simulink model "MotionLab_DigitalTwin"  (R2024b)
settings: Solver=ode3  StartTime=0.0  StopTime=inf  FixedStep=Ts  RelTol=1e-3  AbsTol=1e-3
model workspace: external: MATLAB File .\Parameters.m (data not in the file)
values from neighbouring files (symbols this model uses):
  L2 = 830e-3    (= 0.83)    [Robot_parameters.m]
  L3 = 1160e-3    (= 1.16)    [Robot_parameters.m]
  L4 = 250e-3    (= 0.25)    [Robot_parameters.m]
undefined symbols (not defined in the file or in its folder): smiData, smiDataBig, smiDataBigTop, smiDataRobot, Var, X, Y, Z
libraries: sm_lib x490, nesl_utility x87, slrealtimeutilitieslib x1, slrealtimeiplib x1, aerolibanimutils x1
(part 1 of 15)
settings Model: SimulationMode=accelerator  Creator=thoma  LastModifiedBy=jojoa
settings SolverCC: AutoScaleAbsTol=off  AlgebraicLoopSolver=TrustRegion  MaxZcPerStep=1
settings DebuggingCC: UnconnectedInputMsg=warning  UnconnectedOutputMsg=warning  UnconnectedLineMsg=warning  SymbolicDimsDataTypeCodeGenerationDiagnostic=none
settings ModelReferenceCC: EnableRefExpFcnMdlSchedulingChecks=on
settings SFSimCC: CustomCodeUndefinedFunction=UseInterfaceOnly
settings RTWCC: GPUComputeCapability=3.5  DLArmComputeVersion=19.05
settings SimscapeCC: SimscapeLogType=all  SimscapeLogSimulationStatistics=on  SimscapeLogDataHistory=10000
settings ExplorerConfigSet: InternalSimMechanicsExplorerSettings="<ExplorerConfiguration><canonicalview>default</canonicalview><AnimationSetting><BasePlaybackSpeed>1.0</BasePlaybackSpeed><PlaybackSpeedFactor>1.0</PlaybackSpeedFactor></AnimationSetting><TilePanel><TileInfo><Tiles Columns=\"1\" Count=\"1\" Rows=\"1\"><Column Weight=\"1\"/><Row Weight=\"1\"/><Tile Height=\"1\" Width=\"1\" X=\"0\" Y=\"0\"/></Tiles></TileInfo><SceneInfo><SceneViewer><BGColor><R>1</R><G>1</G><B>1</B></BGColor><Camera><DoPerspective>off</DoPerspective><Position><X>-13.1233061332893666</X><Y>-1.45430535142352291</Y><Z>4.06844865702874081</Z></Position><Center><X>-0.172917730343304044</X><Y>1.29106577544240819</Y><Z>3.17239564313608469</Z></Center><Up><X>0.0683722661013297928</X><Y>0.00309773406366908866</Y><Z>0.997655069285893203</Z></Up><ViewLimDist>1</ViewLimDist><YLim>5.21326136870264634</YLim><XLim>6.07904176706880239</XLim></Camera></SceneViewer></SceneInfo></TilePanel><MechEditorPanel><Cameras/><GfxPanelCameraMap/><VideoCreator><PlaybackSpeedRatio>1.0</PlaybackSpeedRatio><FrameRate>30</FrameRate><VideoFormat>Motion JPEG AVI</VideoFormat><FrameSize>auto</FrameSize></VideoCreator></MechEditorPanel></ExplorerConfiguration>"

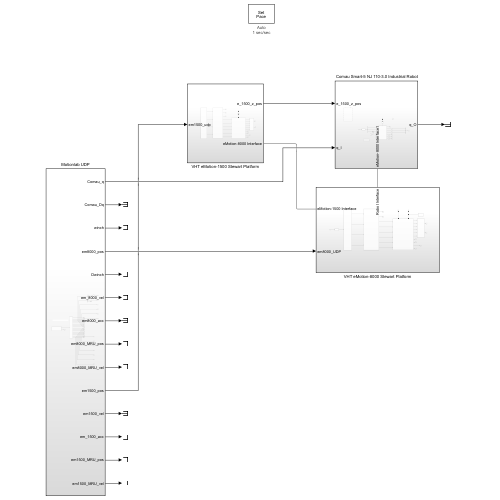
[thumbnail: Simulink's stored preview of the top-level diagram]
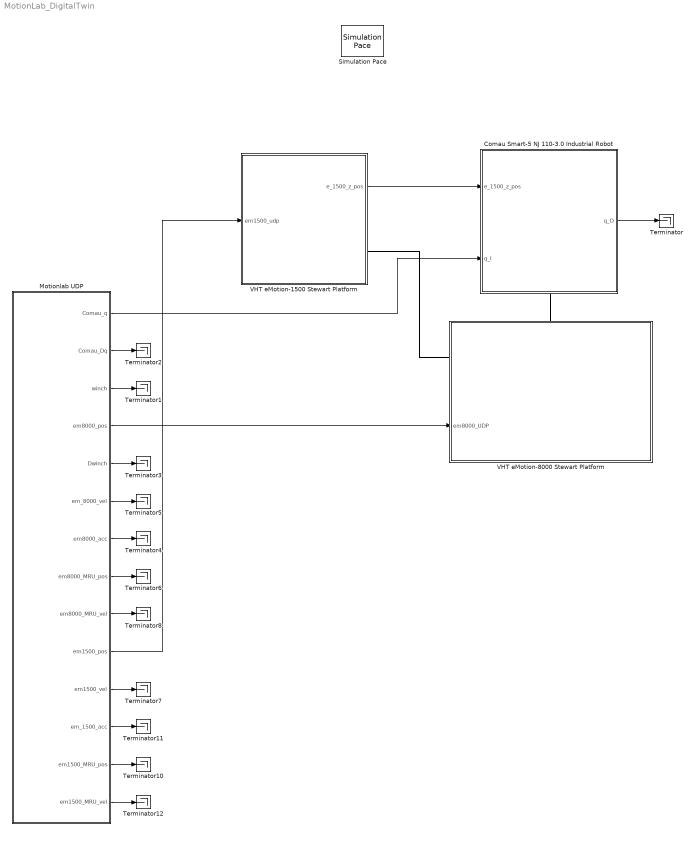
== system MotionLab_DigitalTwin ==
  " Comau Smart-5 NJ 110-3.0 Industrial Robot" : Subsystem
      settings: PortSchema="{\"entries\":[{\"content\":{\"sides\":[{\"content\":{\"connectorIds\":[\"In1\",\"In2\"]},\"type\":\"ConnectorPlacement.EquallySpacedRectSide\",\"uuid\":\"640b4a80-a183-4fda-808f-40bbc59803ff\"},{\"content\":{\"connectorIds\":[\"Out1\"],\"side\":\"RIGHT\"},\"type\":\"ConnectorPlacement.EquallySpacedRectSide\",\"uuid\":\"26bc9ede-0f7e-4968-8fcb-4700031f2d04\"},{\"content\":{\"side\":\"TOP\"},\"type\":\"ConnectorPlacement.EquallySpacedRectSide\",\"uuid\":\"f8c1678d-f904-4b2c-ba65-fdabdde128e7\"},{\"content\":{\"connectorIds\":[\"RConn1\"],\"side\":\"BOTTOM\"},\"type\":\"ConnectorPlacement.EquallySpacedRectSide\",\"uuid\":\"31ccf5cf-cde0-4868-907a-e8310ac905dd\"}]},\"type\":\"ConnectorPlacement.EquallySpacedConnector\",\"uuid\":\"53f72707-ebf3-419b-a015-bfc27a2c6f75\"}],\"packageUris\":[\"http://schema.mathworks.com/mf0/Connector/R2020b\"],\"version\":\"1.0\"}"
  Motionlab UDP : Subsystem
  Simulation Pace : aerolibanimutils/Simulation Pace  SimulationPace=1  SleepMode=Auto  OutputPaceError=off  SampleTime=0.1
  Terminator{,1..8,10..12} (12 alike) : Terminator
  VHT eMotion-1500 Stewart Platform : Subsystem
  VHT eMotion-8000 Stewart Platform : Subsystem
      settings: PortSchema="{\"entries\":[{\"content\":{\"sides\":[{\"content\":{\"connectorIds\":[\"LConn1\",\"In1\"]},\"type\":\"ConnectorPlacement.EquallySpacedRectSide\",\"uuid\":\"db0806e8-caa2-421d-936b-a6f75aa8bfb7\"},{\"content\":{\"side\":\"RIGHT\"},\"type\":\"ConnectorPlacement.EquallySpacedRectSide\",\"uuid\":\"91c2d1eb-1633-461d-b983-e6d74b9ad515\"},{\"content\":{\"connectorIds\":[\"LConn2\"],\"side\":\"TOP\"},\"type\":\"ConnectorPlacement.EquallySpacedRectSide\",\"uuid\":\"8a695272-575a-45c8-aed2-3cc82643c7b5\"}]},\"type\":\"ConnectorPlacement.EquallySpacedConnector\",\"uuid\":\"60269924-cfd7-445e-9c1f-e8fc9453bc0f\"}],\"packageUris\":[\"http://schema.mathworks.com/mf0/Connector/R2020b\"],\"version\":\"1.0\"}"
  wires:
  Motionlab UDP/2(Comau_Dq) -> Terminator2/1
  Motionlab UDP/3(winch) -> Terminator1/1
  VHT eMotion-1500 Stewart Platform/1(e_1500_z_pos) -> " Comau Smart-5 NJ 110-3.0 Industrial Robot"/1(e_1500_z_pos)
  Motionlab UDP/4(em8000_pos) -> VHT eMotion-8000 Stewart Platform/1(em8000_UDP)
  Motionlab UDP/1(Comau_q) -> " Comau Smart-5 NJ 110-3.0 Industrial Robot"/2(q_I)
  Motionlab UDP/14(em1500_MRU_vel) -> Terminator12/1
  Motionlab UDP/13(em1500_MRU_pos) -> Terminator10/1
  Motionlab UDP/12(em_1500_acc) -> Terminator11/1
  Motionlab UDP/11(em1500_vel) -> Terminator7/1
  Motionlab UDP/9(em8000_MRU_vel) -> Terminator8/1
  Motionlab UDP/8(em8000_MRU_pos) -> Terminator6/1
  Motionlab UDP/7(em8000_acc) -> Terminator4/1
  Motionlab UDP/6(em_8000_vel) -> Terminator5/1
  Motionlab UDP/5(Dwinch) -> Terminator3/1
  Motionlab UDP/10(em1500_pos) -> VHT eMotion-1500 Stewart Platform/1(em1500_udp)
  " Comau Smart-5 NJ 110-3.0 Industrial Robot"/1(q_O) -> Terminator/1
  connections:
  VHT eMotion-8000 Stewart Platform/LConn2 -- " Comau Smart-5 NJ 110-3.0 Industrial Robot"/RConn1
  VHT eMotion-1500 Stewart Platform/RConn1 -- VHT eMotion-8000 Stewart Platform/LConn1

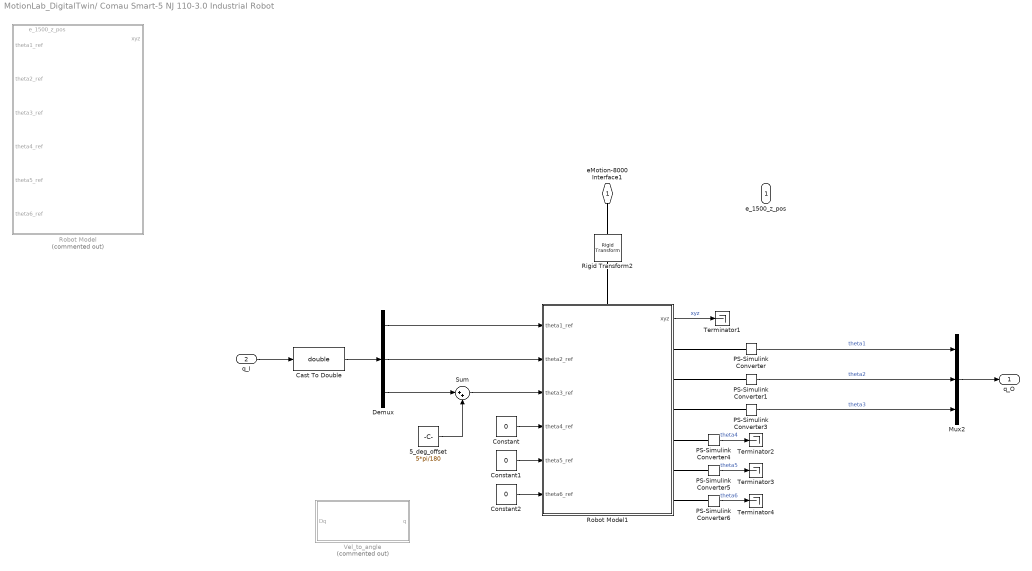
== system MotionLab_DigitalTwin/ Comau Smart-5 NJ 110-3.0 Industrial Robot ==
  e_1500_z_pos : Inport
  q_I : Inport  Port=2
  5_deg_offset : Constant  Value=5*pi/180
  Cast To Double : DataTypeConversion  OutDataTypeStr=double  SaturateOnIntegerOverflow=off  RndMeth=Floor
  Constant : Constant  Value=0
  Constant1 : Constant  Value=0
  Constant2 : Constant  Value=0
  Demux : Demux  Outputs=3
  Mux2 : Mux  Inputs=3
  PS-Simulink Converter{,1,3..6} (6 alike) : nesl_utility/PS-Simulink Converter  PhysicalDomain=network_engine_domain  SubClassName=ps_output  LeftPortType=input  RightPortType=output  PseudoPeriodic=off  Frequencies=[]  VectorFormat=inherit  Unit=inherit  AffineConversion=off
  Rigid Transform2 : sm_lib/Frames and Transforms/Rigid Transform  RotationMethod=StandardAxis  FollAlignAxisA=+X  BaseAlignAxisA=+Y  FollAlignAxisB=+Y  BaseAlignAxisB=+Z  RotationStandardAxis=+Z  RotationAngle=130  RotationAngleUnits=deg  RotationArbitraryAxis=[0 0 1]  RotationSequenceAxes=FollowerAxes  RotationSequence=XYX  RotationSequenceAngles=[0 0 0]  RotationSequenceAnglesUnits=deg  RotationMatrix=[1 0 0; 0 1 0; 0 0 1]  Quaternion=[1 0 0 0]  TranslationMethod=Cartesian  TranslationCartesianOffset=[-1.1 1.8 0]  TranslationCartesianOffsetUnits=m  TranslationStandardAxis=+Z  TranslationStandardOffset=0  TranslationStandardOffsetUnits=m  TranslationROffset=0  TranslationROffsetUnits=m  TranslationThetaOffset=0  TranslationThetaOffsetUnits=deg  TranslationZOffset=0  TranslationZOffsetUnits=m
  Robot Model : Subsystem  Commented=on
      settings: PortSchema="{\"entries\":[{\"content\":{\"sides\":[{\"content\":{\"connectorIds\":[\"In1\",\"In2\",\"In3\",\"In4\",\"In5\",\"In6\"]},\"type\":\"ConnectorPlacement.EquallySpacedRectSide\",\"uuid\":\"596e8081-7d32-40df-b045-1d7fd921636b\"},{\"content\":{\"connectorIds\":[\"Out1\",\"RConn1\",\"RConn2\",\"RConn3\",\"RConn4\",\"RConn5\",\"RConn6\"],\"side\":\"RIGHT\"},\"type\":\"ConnectorPlacement.EquallySpacedRectSide\",\"uuid\":\"d1c0a788-d140-463e-89bf-e77f8fddfed9\"},{\"content\":{\"connectorIds\":[\"In7\",\"LConn1\"],\"side\":\"TOP\"},\"type\":\"ConnectorPlacement.EquallySpacedRectSide\",\"uuid\":\"500a65c5-6d2e-4b69-b3c7-6891d74bdde9\"},{\"content\":{\"side\":\"BOTTOM\"},\"type\":\"ConnectorPlacement.EquallySpacedRectSide\",\"uuid\":\"a9e79246-915d-4b82-96f6-19b412fae044\"}]},\"type\":\"ConnectorPlacement.EquallySpacedConnector\",\"uuid\":\"c6f36c8a-4b47-4d61-838b-5cbf0af5ae4a\"}],\"packageUris\":[\"http://schema.mathworks.com/mf0/Connector/R2020b\"],\"version\":\"1.0\"}"
  Robot Model1 : Subsystem
      settings: PortSchema="{\"entries\":[{\"content\":{\"sides\":[{\"content\":{\"connectorIds\":[\"In1\",\"In2\",\"In3\",\"In4\",\"In5\",\"In6\"]},\"type\":\"ConnectorPlacement.EquallySpacedRectSide\",\"uuid\":\"e1ecbf6a-08a4-4f0e-ba37-ca50bc9b1b85\"},{\"content\":{\"connectorIds\":[\"Out1\",\"RConn1\",\"RConn2\",\"RConn3\",\"RConn4\",\"RConn5\",\"RConn6\"],\"side\":\"RIGHT\"},\"type\":\"ConnectorPlacement.EquallySpacedRectSide\",\"uuid\":\"11387824-9cae-4bb3-bef8-98dd2b653f30\"},{\"content\":{\"connectorIds\":[\"LConn1\"],\"side\":\"TOP\"},\"type\":\"ConnectorPlacement.EquallySpacedRectSide\",\"uuid\":\"e4a96768-bc73-4170-aa82-07a60290a458\"}]},\"type\":\"ConnectorPlacement.EquallySpacedConnector\",\"uuid\":\"0c5d86b4-379e-4c58-9d26-a0c23d78386a\"}],\"packageUris\":[\"http://schema.mathworks.com/mf0/Connector/R2020b\"],\"version\":\"1.0\"}"
  Sum : Sum  Inputs=|++
  Terminator{1..4} (4 alike) : Terminator
  Vel_to_angle : Subsystem  Commented=on
  eMotion-8000 Interface1 : PMIOPort  Side=Right
  q_O : Outport
  wires:
  q_I/1 -> Cast To Double/1
  5_deg_offset/1 -> Sum/2
  Demux/2 -> Robot Model1/2(theta2_ref)
  Demux/1 -> Robot Model1/1(theta1_ref)
  PS-Simulink Converter3/1 -> Mux2/3  "theta3"
  PS-Simulink Converter1/1 -> Mux2/2  "theta2"
  PS-Simulink Converter5/1 -> Terminator3/1  "theta5"
  Constant/1 -> Robot Model1/4(theta4_ref)
  Mux2/1 -> q_O/1
  Constant2/1 -> Robot Model1/6(theta6_ref)
  Constant1/1 -> Robot Model1/5(theta5_ref)
  PS-Simulink Converter6/1 -> Terminator4/1  "theta6"
  PS-Simulink Converter/1 -> Mux2/1  "theta1"
  Demux/3 -> Sum/1
  Sum/1 -> Robot Model1/3(theta3_ref)
  Robot Model1/1(xyz) -> Terminator1/1  "xyz"
  Cast To Double/1 -> Demux/1
  PS-Simulink Converter4/1 -> Terminator2/1  "theta4"
  connections:
  Robot Model1/RConn5 -- PS-Simulink Converter5/LConn1
  Robot Model1/LConn1 -- Rigid Transform2/RConn1
  Robot Model1/RConn3 -- PS-Simulink Converter3/LConn1
  eMotion-8000 Interface1/RConn1 -- Rigid Transform2/LConn1
  Robot Model1/RConn4 -- PS-Simulink Converter4/LConn1
  PS-Simulink Converter/LConn1 -- Robot Model1/RConn1
  Robot Model1/RConn6 -- PS-Simulink Converter6/LConn1
  PS-Simulink Converter1/LConn1 -- Robot Model1/RConn2

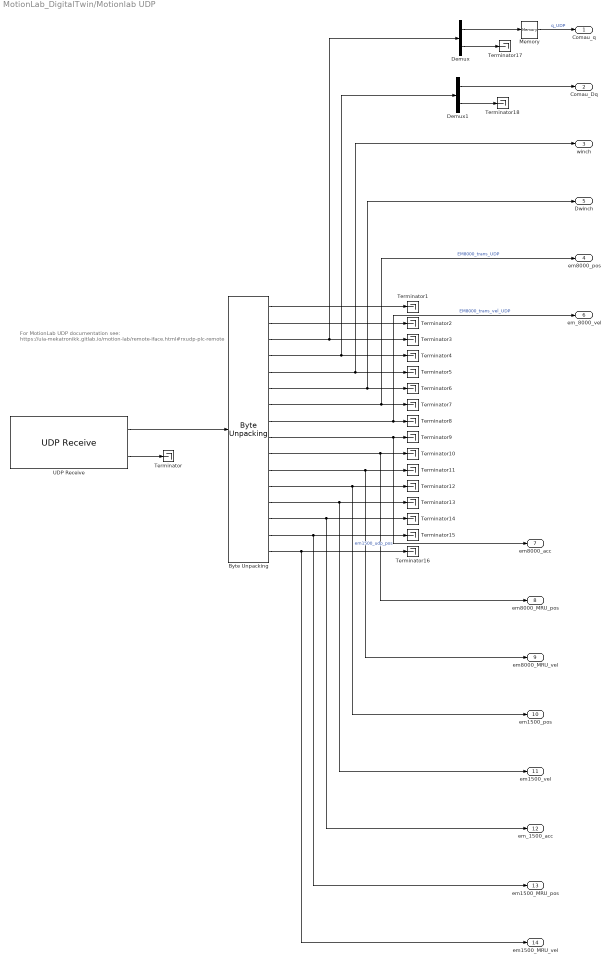
== system MotionLab_DigitalTwin/Motionlab UDP ==
  note: For MotionLab UDP documentation see:
      |  https://uia-mekatronikk.gitlab.io/motion-lab/remote-iface.html#rxudp-plc-remote
  Byte Unpacking : slrealtimeutilitieslib/Byte Unpacking  MaskUnpackedDataTypes={'uint32', 'single', 'single', 'single', 'single', 'single', 'single', 'single', 'single', 'single', 'single', 'single', 'single', 'single', 'single', 'single'}  MaskUnpackedDataSizes={[1], [1], [6], [6], [1], [1], [6], [6], [6], [6], [6], [6], [6], [6], [6], [6]}  MaskAlignment=1
  Demux : Demux  Outputs=2
  Demux1 : Demux  Outputs=2
  Memory : Memory  InitialCondition=[0 0 -1.57]
  Terminator{,1..18} (19 alike) : Terminator
  UDP Receive : slrealtimeiplib/UDP Receive  useHostTargetConn=on  ipAddress=10.10.10.15  localPort=50060  rcvWidth=304  rcvFmAny=on  fmAddress='10.10.10.10'  sampleTime=Ts  enableMessage=off  maxPackets=1
  Comau_q : Outport
  Comau_Dq : Outport  Port=2
  winch : Outport  Port=3
  em8000_pos : Outport  Port=4
  Dwinch : Outport  Port=5
  em_8000_vel : Outport  Port=6
  em8000_acc : Outport  Port=7
  em8000_MRU_pos : Outport  Port=8
  em8000_MRU_vel : Outport  Port=9
  em1500_pos : Outport  Port=10
  em1500_vel : Outport  Port=11
  em_1500_acc : Outport  Port=12
  em1500_MRU_pos : Outport  Port=13
  em1500_MRU_vel : Outport  Port=14
  wires:
  UDP Receive/1 -> Byte Unpacking/1
  UDP Receive/2 -> Terminator/1
  Byte Unpacking/1 -> Terminator1/1
  Byte Unpacking/2 -> Terminator2/1
  Byte Unpacking/3 -> Terminator3/1, Demux/1
  Byte Unpacking/4 -> Terminator4/1, Demux1/1
  Byte Unpacking/5 -> Terminator5/1, winch/1
  Byte Unpacking/6 -> Dwinch/1, Terminator6/1
  Byte Unpacking/7 -> em8000_pos/1, Terminator7/1  "EM8000_trans_UDP"
  Byte Unpacking/8 -> em_8000_vel/1, Terminator8/1  "EM8000_trans_vel_UDP"
  Byte Unpacking/9 -> em8000_acc/1, Terminator9/1
  Byte Unpacking/10 -> Terminator10/1, em8000_MRU_pos/1
  Byte Unpacking/11 -> Terminator11/1, em8000_MRU_vel/1
  Byte Unpacking/12 -> Terminator12/1, em1500_pos/1  "em1500_udp_pos"
  Byte Unpacking/13 -> Terminator13/1, em1500_vel/1
  Byte Unpacking/14 -> Terminator14/1, em_1500_acc/1
  Byte Unpacking/15 -> em1500_MRU_pos/1, Terminator15/1
  Byte Unpacking/16 -> em1500_MRU_vel/1, Terminator16/1
  Demux/1 -> Memory/1
  Demux/2 -> Terminator17/1
  Memory/1 -> Comau_q/1  "q_UDP"
  Demux1/1 -> Comau_Dq/1
  Demux1/2 -> Terminator18/1

== system MotionLab_DigitalTwin/VHT eMotion-1500 Stewart Platform ==
  em1500_udp : Inport
  ExtractAndCombinePosAndVel1 : Subsystem
  Inverse Kinematics : Subsystem
  Motion Generator : Subsystem
  Rigid Transform : sm_lib/Frames and Transforms/Rigid Transform  RotationMethod=None  FollAlignAxisA=+X  BaseAlignAxisA=+Y  FollAlignAxisB=+Y  BaseAlignAxisB=+Z  RotationStandardAxis=+Z  RotationAngle=0.0  RotationAngleUnits=deg  RotationArbitraryAxis=[0 0 1]  RotationSequenceAxes=FollowerAxes  RotationSequence=XYX  RotationSequenceAngles=[0 0 0]  RotationSequenceAnglesUnits=deg  RotationMatrix=[1 0 0; 0 1 0; 0 0 1]  Quaternion=[1 0 0 0]  TranslationMethod=Cartesian  TranslationCartesianOffset=[-3 4 0]  TranslationCartesianOffsetUnits=m  TranslationStandardAxis=+Z  TranslationStandardOffset=0  TranslationStandardOffsetUnits=m  TranslationROffset=0  TranslationROffsetUnits=m  TranslationThetaOffset=0  TranslationThetaOffsetUnits=deg  TranslationZOffset=0  TranslationZOffsetUnits=m
  Terminator{,1..7} (8 alike) : Terminator
  UiA Stewart Platform1 : Subsystem
      settings: PortSchema="{\"entries\":[{\"content\":{\"sides\":[{\"content\":{\"connectorIds\":[\"In1\",\"In2\",\"In3\",\"In4\",\"In5\",\"In6\"]},\"type\":\"ConnectorPlacement.EquallySpacedRectSide\",\"uuid\":\"7f0ff7fd-0348-45ad-beb9-8ad2ec3e2887\"},{\"content\":{\"connectorIds\":[\"Out1\",\"Out2\",\"Out3\",\"Out4\",\"Out5\",\"Out6\",\"Out7\",\"Out8\",\"Out9\",\"Out10\"],\"side\":\"RIGHT\"},\"type\":\"ConnectorPlacement.EquallySpacedRectSide\",\"uuid\":\"276042a1-7937-4cae-810e-b80b5f2637b1\"},{\"content\":{\"connectorIds\":[\"LConn1\"],\"side\":\"TOP\"},\"type\":\"ConnectorPlacement.EquallySpacedRectSide\",\"uuid\":\"d74fb182-1c8f-4c06-a6da-c93034697881\"}]},\"type\":\"ConnectorPlacement.EquallySpacedConnector\",\"uuid\":\"3d2973ff-43c5-4cbf-9014-0a5cde3717a6\"}],\"packageUris\":[\"http://schema.mathworks.com/mf0/Connector/R2020b\"],\"version\":\"1.0\"}"
  eMotion-8000 Interface : PMIOPort  Side=Right
  e_1500_z_pos : Outport
  wires:
  UiA Stewart Platform1/1("xCyl1, vCyl1, fCyl1") -> ExtractAndCombinePosAndVel1/1(In1)
  UiA Stewart Platform1/6("xCyl6, vCyl6, fCyl6") -> ExtractAndCombinePosAndVel1/6(In6)
  UiA Stewart Platform1/7(R) -> Terminator/1
  UiA Stewart Platform1/3("xCyl3, vCyl3, fCyl3") -> ExtractAndCombinePosAndVel1/3(In3)
  UiA Stewart Platform1/8(w) -> Terminator1/1
  UiA Stewart Platform1/4("xCyl4, vCyl4, fCyl4") -> ExtractAndCombinePosAndVel1/4(In4)
  UiA Stewart Platform1/10(v) -> Terminator5/1
  UiA Stewart Platform1/9(p) -> Terminator2/1  "em1500_model_pos"
  UiA Stewart Platform1/2("xCyl2, vCyl2, fCyl2") -> ExtractAndCombinePosAndVel1/2(In2)
  UiA Stewart Platform1/5("xCyl5, vCyl5, fCyl5") -> ExtractAndCombinePosAndVel1/5(In5)
  Inverse Kinematics/2(y1) -> Terminator3/1
  ExtractAndCombinePosAndVel1/2(ActualLegVel) -> Terminator4/1
  ExtractAndCombinePosAndVel1/1(ActualLegPos) -> Terminator6/1
  Motion Generator/4(v_top) -> Inverse Kinematics/4(vel)
  Motion Generator/1(R_top) -> Inverse Kinematics/1(Rot)
  Motion Generator/2(w_top) -> Inverse Kinematics/2(w)
  Motion Generator/3(ptop) -> Inverse Kinematics/3(pos)
  Inverse Kinematics/3(e_1500_z_pos) -> e_1500_z_pos/1
  Inverse Kinematics/1(y) -> Terminator7/1  "em1500_y"
  Inverse Kinematics/4(xRefCyl1) -> UiA Stewart Platform1/1(xRefCyl1)
  Inverse Kinematics/5(xRefCyl2) -> UiA Stewart Platform1/2(xRefCyl2)
  Inverse Kinematics/6(xRefCyl3) -> UiA Stewart Platform1/3(xRefCyl3)
  Inverse Kinematics/7(xRefCyl4) -> UiA Stewart Platform1/4(xRefCyl4)
  Inverse Kinematics/8(xRefCyl5) -> UiA Stewart Platform1/5(xRefCyl5)
  Inverse Kinematics/9(xRefCyl6) -> UiA Stewart Platform1/6(xRefCyl6)
  em1500_udp/1 -> Motion Generator/1(em1500_udp)
  connections:
  Rigid Transform/RConn1 -- UiA Stewart Platform1/LConn1
  eMotion-8000 Interface/RConn1 -- Rigid Transform/LConn1

== system MotionLab_DigitalTwin/VHT eMotion-8000 Stewart Platform ==
  em8000_UDP : Inport
  Cast To Double : DataTypeConversion  OutDataTypeStr=double  SaturateOnIntegerOverflow=off  RndMeth=Floor
  ExtractAndCombinePosAndVel : Subsystem
  Inverse Kinematics : Subsystem
  MBS Config : Subsystem
  Motion Control System : Subsystem
  Terminator{,1..7} (8 alike) : Terminator
  UiA Stewart Platform : Subsystem
      settings: PortSchema="{\"entries\":[{\"content\":{\"sides\":[{\"content\":{\"connectorIds\":[\"In1\",\"In2\",\"In3\",\"In4\",\"In5\",\"In6\"]},\"type\":\"ConnectorPlacement.EquallySpacedRectSide\",\"uuid\":\"de8fd662-7a9e-4209-b357-dad0c75e3639\"},{\"content\":{\"connectorIds\":[\"Out1\",\"Out2\",\"Out3\",\"Out4\",\"Out5\",\"Out6\",\"Out7\",\"Out8\",\"Out9\",\"Out10\"],\"side\":\"RIGHT\"},\"type\":\"ConnectorPlacement.EquallySpacedRectSide\",\"uuid\":\"e834d12e-6262-442b-ab59-0eaa631772a0\"},{\"content\":{\"connectorIds\":[\"LConn1\",\"LConn2\"],\"side\":\"TOP\"},\"type\":\"ConnectorPlacement.EquallySpacedRectSide\",\"uuid\":\"a8020181-8251-4e51-94b7-b1fc3bb6a903\"}]},\"type\":\"ConnectorPlacement.EquallySpacedConnector\",\"uuid\":\"4c8cdd83-1355-404f-82e4-691ae5a3080a\"}],\"packageUris\":[\"http://schema.mathworks.com/mf0/Connector/R2020b\"],\"version\":\"1.0\"}"
  eMotion-1500 Interface : PMIOPort  Side=Left
  Robot Interface : PMIOPort  Port=2  Side=Left
  wires:
  Motion Control System/3(ptop) -> Inverse Kinematics/3(posBig)
  Motion Control System/4(v_top) -> Inverse Kinematics/4(velBig)
  UiA Stewart Platform/9(pBig) -> Terminator4/1  "em8000_model_pos"
  UiA Stewart Platform/4("xCyl4, vCyl4, fCyl1") -> ExtractAndCombinePosAndVel/4(In4)
  UiA Stewart Platform/7(RBig) -> Terminator/1
  UiA Stewart Platform/10(vBig) -> Terminator5/1
  UiA Stewart Platform/8(wBig) -> Terminator3/1
  Motion Control System/1(R_top) -> Inverse Kinematics/1(RotBig)
  UiA Stewart Platform/6("xCyl6, vCyl6, fCyl1") -> ExtractAndCombinePosAndVel/6(In6)
  Motion Control System/2(w_top) -> Inverse Kinematics/2(wBig)
  UiA Stewart Platform/1("xCyl1, vCyl1, fCyl2") -> ExtractAndCombinePosAndVel/1(In1)
  UiA Stewart Platform/2("xCyl2, vCyl2, fCyl1") -> ExtractAndCombinePosAndVel/2(In2)
  UiA Stewart Platform/3("xCyl3, vCyl3, fCyl1") -> ExtractAndCombinePosAndVel/3(In3)
  UiA Stewart Platform/5("xCyl5, vCyl5, fCyl1") -> ExtractAndCombinePosAndVel/5(In5)
  Inverse Kinematics/2(y1) -> Terminator1/1
  ExtractAndCombinePosAndVel/2(ActualLegVel) -> Terminator2/1
  ExtractAndCombinePosAndVel/1(ActualLegPos) -> Terminator6/1
  Inverse Kinematics/1(y) -> Terminator7/1
  Inverse Kinematics/3(xRefCyl1) -> UiA Stewart Platform/1(xRefCyl1)
  Inverse Kinematics/4(xRefCyl2) -> UiA Stewart Platform/2(xRefCyl2)
  Inverse Kinematics/5(xRefCyl3) -> UiA Stewart Platform/3(xRefCyl3)
  Inverse Kinematics/6(xRefCyl4) -> UiA Stewart Platform/4(xRefCyl4)
  Inverse Kinematics/7(xRefCyl5) -> UiA Stewart Platform/5(xRefCyl5)
  Inverse Kinematics/8(xRefCyl6) -> UiA Stewart Platform/6(xRefCyl6)
  em8000_UDP/1 -> Cast To Double/1
  Cast To Double/1 -> Motion Control System/1(em8000_UDP)
  connections:
  Robot Interface/RConn1 -- UiA Stewart Platform/LConn1
  eMotion-1500 Interface/RConn1 -- MBS Config/RConn1 -- UiA Stewart Platform/LConn2
